simulink model "gocart_simulink"  (R2018a)
settings: Solver=VariableStepAuto  StartTime=0.0  StopTime=10.0  MaxStep=0.2  RelTol=1e-4
values from neighbouring files (symbols this model uses):
  T_f = 1    [gocart_matlab.m]
undefined symbols (not defined in the file or in its folder): sigbuilder_block
libraries: powerlib x3
settings Model: Creator=prettibon  LastModifiedBy=prettibon
settings CodeAppCC: StateflowObjectComments=on

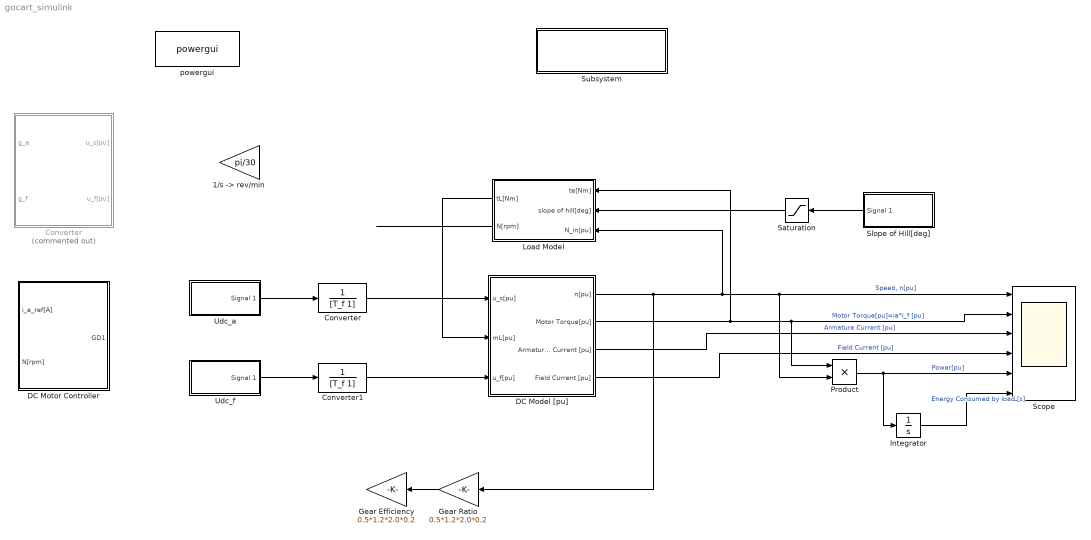
== system gocart_simulink ==
  "1/s -> rev/min" : Gain  Gain=pi/30
  Converter : TransferFcn  Denominator=[T_f 1]
  "Converter " : Subsystem  Commented=on
      mask DialogControl DescGroupVar Prompt: %<1>
  Converter1 : TransferFcn  Denominator=[T_f 1]
  DC Model [pu] : Subsystem  mask{ra=0.29, la=2.612e-3, Tm=1.768, Tf=1, Me=0, Ohmega=0, Eff=0}
      mask prompts: ra "Armature resistance [pu]"; la "Armature inductance [pu]"; Tm "Mechanical time constant [s]"; Tf "Field time constant [s]"; Me "Torque Basis [Nm]"; Ohmega "Speed Basis [1/s]"; Eff "Efficiency of Motor [%]"
      mask DialogControl Container3 Prompt: For Gear Box
  DC Motor Controller : Subsystem
      mask DialogControl DescGroupVar Prompt: %<1>
  "Gear Efficiency " : Gain  Gain=0.5*1.2*2.0*0.2
  "Gear Ratio " : Gain  Gain=0.5*1.2*2.0*0.2
  Integrator : Integrator
  "Load Model " : Subsystem  mask{rho=1.2, c_d=0.2, A=2, j_m=1, g=9.81, m=200, mu_r=0.01}
      mask prompts: rho "Air density"; c_d "Drag coefficient"; A "Area of cart"; j_m "Motor inertia"; g "Gravity"; m "Mass of gocart"; mu_r "Wheel resistance coefficient"
  Product : Product
  Saturation : Saturate  UpperLimit=20  LowerLimit=-20
  Scope : Scope  NumInputPorts=6
  Slope of Hill[deg] : Subsystem  Tag=STV Subsys  LoadFcn=sigbuilder_block('load');  StartFcn=sigbuilder_block('start');  StopFcn=sigbuilder_block('stop');  ClipboardFcn=sigbuilder_block('clipboard');  mask(Sigbuilder block){tuvar=[0:10]}
      mask help: Simulink:masks:SigbuilderBlock_MD
      mask init:
      | if ~strcmp(get_param(bdroot(gcbh),'SimulationStatus'),'stopped') tuvar = sigbuilder_block('maskInit'); end
      settings: CopyFcn=sigbuilder_block('copy');  DeleteFcn=sigbuilder_block('delete');  ModelCloseFcn=sigbuilder_block('modelClose');  PreSaveFcn=sigbuilder_block('preSave');  PauseFcn=sigbuilder_block('pause');  ContinueFcn=sigbuilder_block('continue');  NameChangeFcn=sigbuilder_block('namechange');  OpenFcn=sigbuilder_block('open',[5.5 5.5 949 474.5 ]);  CloseFcn=sigbuilder_block('close');
      mask Display: plot(0, 0, 100, 100,[2, 2, 32, 32, 2], [68, 8, 8, 68, 68],[32, 2], [38, 38], [32, 19, 2],[53, 60, 44], [32, 17, 17, 2],[16, 16, 31, 31]);txt = getActiveGroup(gcbh);text(2, 100, txt,'verticalAlignment', 'top');
  Subsystem : Subsystem
      settings: OpenFcn=open_system('power_new_palette')
      mask Display: disp(sprintf('Open Simscape Power Systems\n(Specialized Technology)\nPalette Library'));
  Udc_a : Subsystem  Tag=STV Subsys  LoadFcn=sigbuilder_block('load');  StartFcn=sigbuilder_block('start');  StopFcn=sigbuilder_block('stop');  ClipboardFcn=sigbuilder_block('clipboard');  mask(Sigbuilder block){tuvar=[0:10]}
      mask help: Simulink:masks:SigbuilderBlock_MD
      mask init:
      | if ~strcmp(get_param(bdroot(gcbh),'SimulationStatus'),'stopped') tuvar = sigbuilder_block('maskInit'); end
      settings: CopyFcn=sigbuilder_block('copy');  DeleteFcn=sigbuilder_block('delete');  ModelCloseFcn=sigbuilder_block('modelClose');  PreSaveFcn=sigbuilder_block('preSave');  PauseFcn=sigbuilder_block('pause');  ContinueFcn=sigbuilder_block('continue');  NameChangeFcn=sigbuilder_block('namechange');  OpenFcn=sigbuilder_block('open',[5.5 5.5 949 474.5 ]);  CloseFcn=sigbuilder_block('close');
      mask Display: plot(0, 0, 100, 100,[2, 2, 32, 32, 2], [68, 8, 8, 68, 68],[32, 2], [38, 38], [32, 19, 2],[53, 60, 44], [32, 17, 17, 2],[16, 16, 31, 31]);txt = getActiveGroup(gcbh);text(2, 100, txt,'verticalAlignment', 'top');
  Udc_f : Subsystem  Tag=STV Subsys  LoadFcn=sigbuilder_block('load');  StartFcn=sigbuilder_block('start');  StopFcn=sigbuilder_block('stop');  ClipboardFcn=sigbuilder_block('clipboard');  mask(Sigbuilder block){tuvar=[0:10]}
      mask help: Simulink:masks:SigbuilderBlock_MD
      mask init:
      | if ~strcmp(get_param(bdroot(gcbh),'SimulationStatus'),'stopped') tuvar = sigbuilder_block('maskInit'); end
      settings: CopyFcn=sigbuilder_block('copy');  DeleteFcn=sigbuilder_block('delete');  ModelCloseFcn=sigbuilder_block('modelClose');  PreSaveFcn=sigbuilder_block('preSave');  PauseFcn=sigbuilder_block('pause');  ContinueFcn=sigbuilder_block('continue');  NameChangeFcn=sigbuilder_block('namechange');  OpenFcn=sigbuilder_block('open',[5.5 5.5 949 474.5 ]);  CloseFcn=sigbuilder_block('close');
      mask Display: plot(0, 0, 100, 100,[2, 2, 32, 32, 2], [68, 8, 8, 68, 68],[32, 2], [38, 38], [32, 19, 2],[53, 60, 44], [32, 17, 17, 2],[16, 16, 31, 31]);txt = getActiveGroup(gcbh);text(2, 100, txt,'verticalAlignment', 'top');
  powergui : powerlib/powergui  Priority=1  SimulationMode=Continuous  SampleTime=50e-6  frequency=60  Iterations=50  frequencyindice=0  Pbase=100e6  ErrMax=1e-4  UnitsV=kV  UnitsW=MW  buscounter=0  FunctionMessages=off  echomessages=off  EnableUseOfTLC=off  CurrentSourceSwitches=off  DisableSnubberDevices=off  DisableRonSwitches=off  DisableVfSwitches=off  DisplayEquations=off  SolverType=Tustin/Backward Euler (TBE)  Interpol=off  ExternalGateDelay=off  methode=off  Ts=100  x0status=blocks  SPID=on  SwTol=0  HookPort=off  RestoreLinks=warning  ResistiveCurrentMeasurement=off  Frange=[0:2:500]  Ylog=off  Xlog=on  ShowGrid=off  save=off  variable=ZData  structure=0  ZoomFFT=off  StartTime=0.0  cycles=1  DisplayStyle=1  fundamental=60  FreqAxis=off  MaxFrequency=1000  frequencyindicesteady=1  RmsSteady=1  display=off
  wires:
  DC Model [pu]/4(Field Current [pu]) -> Scope/4  "Field Current [pu]"
  DC Model [pu]/3(Armature Current [pu]) -> Scope/3  "Armature Current [pu]"
  Integrator/1 -> Scope/6  "Energy Consumed by load [s]"
  Product/1 -> Integrator/1, Scope/5  "Power[pu]"
  DC Model [pu]/1(n[pu]) -> "Gear Ratio "/1, Product/2, Scope/1, "Load Model "/3(N_in[pu])  "Speed, n[pu]"
  DC Model [pu]/2(Motor Torque[pu]) -> "Load Model "/1(te[Nm]), Scope/2, Product/1  "Motor Torque[pu]=ia*i_f [pu]"
  "Gear Ratio "/1 -> "Gear Efficiency "/1
  "Load Model "/1(tL[Nm]) -> DC Model [pu]/2(mL[pu])
  Converter/1 -> DC Model [pu]/1(u_s[pu])
  Udc_a/1(Signal 1) -> Converter/1
  Udc_f/1(Signal 1) -> Converter1/1
  Converter1/1 -> DC Model [pu]/3(u_f[pu])
  Slope of Hill[deg]/1(Signal 1) -> Saturation/1
  Saturation/1 -> "Load Model "/2(slope of hill[deg])
  "Load Model "/2(N[rpm]) -> ?

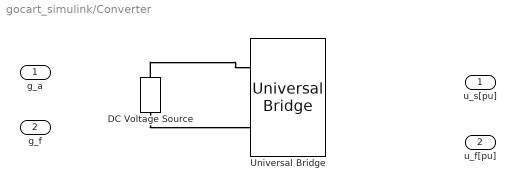
== system gocart_simulink/Converter  ==
  g_a : Inport
  g_f : Inport  Port=2
  DC Voltage Source : powerlib/Electrical Sources/DC Voltage Source  Amplitude=24  Measurements=None
  Universal Bridge : powerlib/Power Electronics/Universal Bridge  Arms=3  SnubberResistance=1e5  SnubberCapacitance=inf  Device=Thyristors  Ron=1e-3  Lon=0  ForwardVoltages="[  0  0  ]"  ForwardVoltage=0  GTOparameters=[ 10e-6 , 20e-6 ]  IGBTparameters=[ 1e-6 , 2e-6 ]  Measurements=None  Measurements_2=None  converterType=Rectifier
  u_s[pu] : Outport
  u_f[pu] : Outport  Port=2
  connections:
  DC Voltage Source/LConn1 -- Universal Bridge/RConn2
  DC Voltage Source/RConn1 -- Universal Bridge/RConn1

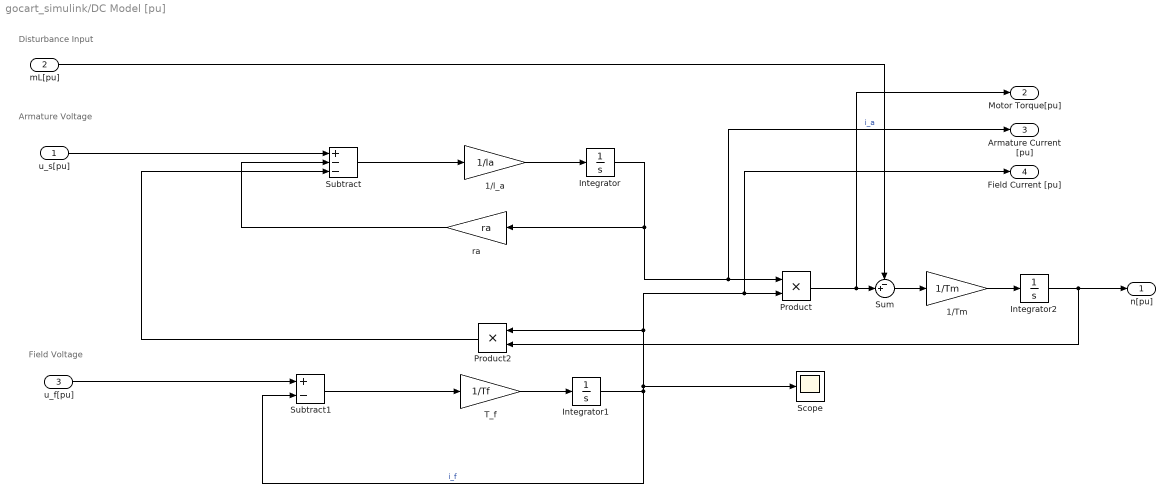
== system gocart_simulink/DC Model [pu] ==
  note: Field Voltage
  note: Armature Voltage
  note: Disturbance Input
  u_s[pu] : Inport
  mL[pu] : Inport  Port=2
  u_f[pu] : Inport  Port=3
  "1/Tm " : Gain  Gain=1/Tm
  "1/l_a " : Gain  Gain=1/la
  Integrator : Integrator
  Integrator1 : Integrator
  Integrator2 : Integrator
  Product : Product
  Product2 : Product
  Scope : Scope
  Subtract : Sum  Inputs=+--
  Subtract1 : Sum  Inputs=+-
  Sum : Sum  Inputs=-+|
  T_f : Gain  Gain=1/Tf
  ra : Gain  Gain=ra
  n[pu] : Outport
  Motor Torque[pu] : Outport  Port=2
  Armature Current [pu] : Outport  Port=3
  Field Current [pu] : Outport  Port=4
  wires:
  mL[pu]/1 -> Sum/1
  Integrator2/1 -> n[pu]/1, Product2/2
  "1/Tm "/1 -> Integrator2/1
  Product2/1 -> Subtract/3
  T_f/1 -> Integrator1/1
  Integrator1/1 -> Product2/1, Product/2, Field Current [pu]/1, Scope/1, Subtract1/2  "i_f"
  u_s[pu]/1 -> Subtract/1
  Subtract/1 -> "1/l_a "/1
  Sum/1 -> "1/Tm "/1
  u_f[pu]/1 -> Subtract1/1
  Integrator/1 -> Armature Current [pu]/1, Product/1, ra/1  "i_a"
  Subtract1/1 -> T_f/1
  "1/l_a "/1 -> Integrator/1
  Product/1 -> Motor Torque[pu]/1, Sum/2
  ra/1 -> Subtract/2

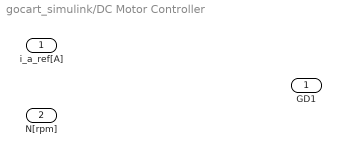
== system gocart_simulink/DC Motor Controller ==
  i_a_ref[A] : Inport
  N[rpm] : Inport  Port=2
  GD1 : Outport

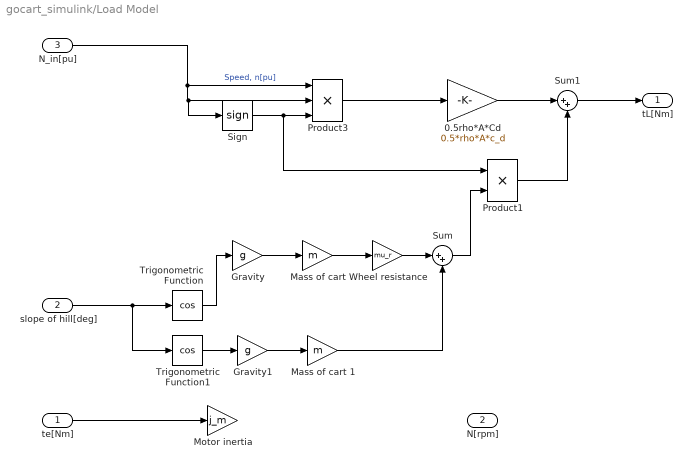
== system gocart_simulink/Load Model  ==
  te[Nm] : Inport
  slope of hill[deg] : Inport  Port=2
  N_in[pu] : Inport  Port=3
  0.5rho*A*Cd : Gain  Gain=0.5*rho*A*c_d
  Gravity : Gain  Gain=g
  Gravity1 : Gain  Gain=g
  "Mass of cart " : Gain  Gain=m
  Mass of cart 1 : Gain  Gain=m
  Motor inertia : Gain  Gain=j_m
  Product1 : Product
  Product3 : Product  Inputs=3
  Sign : Signum
  Sum : Sum  Inputs=|++
  Sum1 : Sum  Inputs=|++
  Trigonometric Function : Trigonometry  Operator=cos
  Trigonometric Function1 : Trigonometry  Operator=cos
  "Wheel resistance " : Gain  Gain=mu_r
  tL[Nm] : Outport
  N[rpm] : Outport  Port=2
  wires:
  N_in[pu]/1 -> Sign/1, Product3/2, Product3/1  "Speed, n[pu]"
  slope of hill[deg]/1 -> Trigonometric Function1/1, Trigonometric Function/1
  Trigonometric Function/1 -> Gravity/1
  Gravity/1 -> "Mass of cart "/1
  Sign/1 -> Product1/1, Product3/3
  "Mass of cart "/1 -> "Wheel resistance "/1
  Sum/1 -> Product1/2
  Product3/1 -> 0.5rho*A*Cd/1
  0.5rho*A*Cd/1 -> Sum1/1
  Sum1/1 -> tL[Nm]/1
  Product1/1 -> Sum1/2
  "Wheel resistance "/1 -> Sum/1
  Trigonometric Function1/1 -> Gravity1/1
  Gravity1/1 -> Mass of cart 1/1
  Mass of cart 1/1 -> Sum/2
  te[Nm]/1 -> Motor inertia/1

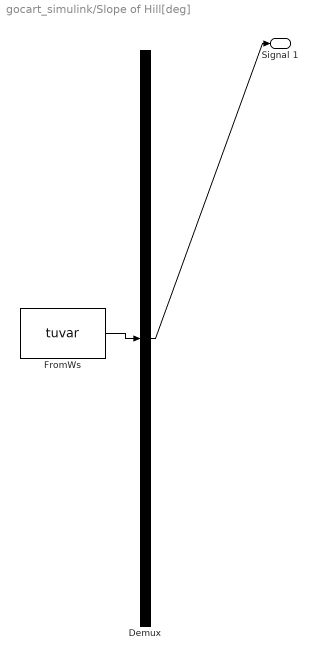
== system gocart_simulink/Slope of Hill[deg] ==
  Demux : Demux  Tag=STV Demux  Outputs=1
  FromWs : FromWorkspace  Tag=STV FromWs  VariableName=tuvar  SampleTime=0
      SigBuilderData=|
      | common.afterFinalStr = 'Extrapolate'
      | common.sampleTime = 0
      | dataSet.timeRange = [0 200]
      | dataSet.name = 'Group 1'
      | sbobj.Groups.Name = 'Group 1'
      | sbobj.Groups.Signals.Name = 'Signal 1'
      | sbobj.Groups.Signals.XData = [0 20.4 80.4 110.6 200]
      | sbobj.Groups.Signals.YData = [0.425 30 0.1 -30 0.425]
      | sbobj.Groups.TimeRange = [0 200]
  Signal 1 : Outport  Tag=STV Outport
  wires:
  FromWs/1 -> Demux/1
  Demux/1 -> Signal 1/1

== system gocart_simulink/Subsystem ==

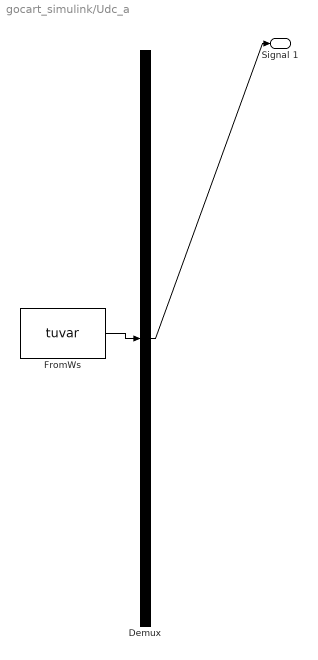
== system gocart_simulink/Udc_a ==
  Demux : Demux  Tag=STV Demux  Outputs=1
  FromWs : FromWorkspace  Tag=STV FromWs  VariableName=tuvar  SampleTime=0
      SigBuilderData=|
      | common.afterFinalStr = 'Extrapolate'
      | common.sampleTime = 0
      | dataSet.timeRange = [0 200]
      | dataSet.name = 'Group 1'
      | sbobj.Groups.Name = 'Group 1'
      | sbobj.Groups.Signals.Name = 'Signal 1'
      | sbobj.Groups.Signals.XData = [0 200]
      | sbobj.Groups.Signals.YData = [0.425 0.425]
      | sbobj.Groups.TimeRange = [0 200]
  Signal 1 : Outport  Tag=STV Outport
  wires:
  FromWs/1 -> Demux/1
  Demux/1 -> Signal 1/1

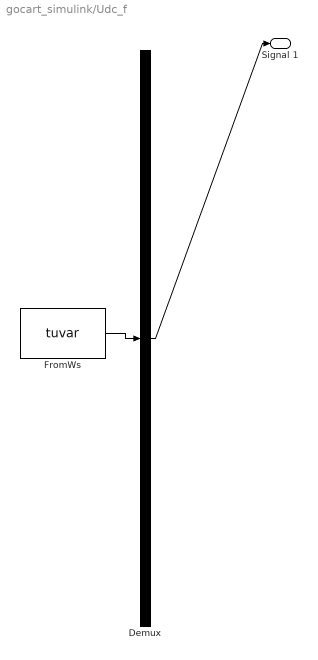
== system gocart_simulink/Udc_f ==
  Demux : Demux  Tag=STV Demux  Outputs=1
  FromWs : FromWorkspace  Tag=STV FromWs  VariableName=tuvar  SampleTime=0
      SigBuilderData=|
      | common.afterFinalStr = 'Extrapolate'
      | common.sampleTime = 0
      | dataSet.timeRange = [0 200]
      | dataSet.name = 'Group 1'
      | sbobj.Groups.Name = 'Group 1'
      | sbobj.Groups.Signals.Name = 'Signal 1'
      | sbobj.Groups.Signals.XData = [0 200]
      | sbobj.Groups.Signals.YData = [0.425 0.425]
      | sbobj.Groups.TimeRange = [0 200]
  Signal 1 : Outport  Tag=STV Outport
  wires:
  FromWs/1 -> Demux/1
  Demux/1 -> Signal 1/1
